simulink model "L0702"  (Simulink 9.1)
settings: Solver=VariableStepAuto  StartTime=0.0  StopTime=10.0  RelTol=1e-3
settings Model: Creator=Asus  LastModifiedBy=Asus
settings DataIOCC: SaveFormat=Dataset
settings OptimizationCC: LifeSpan=auto
settings DebuggingCC: UnderspecifiedInitializationDetection=Simplified  MergeDetectMultiDrivingBlocksExec=error  SFUnexpectedBacktrackingDiag=error  SFNoUnconditionalDefaultTransitionDiag=error  SFExecutionAtInitializationDiag=warning
settings HardwareCC: ProdBitPerPointer=64  ProdBitPerSizeT=64  ProdBitPerPtrDiffT=64  ProdLargestAtomicFloat=Float  ProdIntDivRoundTo=Zero  ProdEndianess=LittleEndian  ProdWordSize=64  ProdHWDeviceType=Intel->x86-64 (Windows64)
settings ModelReferenceCC: PropagateSignalLabelsOutOfModel=on
settings CodeAppCC: StateflowObjectComments=off
settings GRTTargetCC: TargetLangStandard=C99 (ISO)  CombineOutputUpdateFcns=on  GRTInterface=off
settings ConfigComp: CovMetricSettings=dwe  CovHtmlReporting=off  CovSaveCumulativeToWorkspaceVar=off  CovSaveSingleToWorkspaceVar=off  CovExternalEMLEnable=on

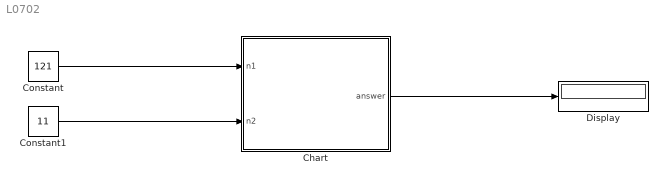
== system L0702 ==
  Chart : Stateflow chart  TreatAsAtomicUnit=on
  Constant : Constant  Value=121
  Constant1 : Constant  Value=11
  Display : Display
  wires:
  Constant1/1 -> Chart/2(n2)
  Constant/1 -> Chart/1(n1)
  Chart/1(answer) -> Display/1

== stateflow chart Chart ==
  state answer
  (default) -> (junction 9) : {N1=n1,N2=n2}
  (junction 9) -> (junction 10) [order 1] : [N1<N2]{N2=N2-N1}
  (junction 9) -> answer [order 3] : {answer=N1}
  (junction 10) -> (junction 9)
  (junction 9) -> (junction 11) [order 2] : [N2<N1]{N1=N1-N2}
  (junction 11) -> (junction 9)
  data: n1 input double; n2 input double; answer output double; N1 local double; N2 local double
